simulink model "AOCS system"  (R2023b)
settings: Solver=ode4  StartTime=0.0  StopTime=1000  FixedStep=0.01  RelTol=1e-3
undefined symbols (not defined in the file): A_e, ARW, e_sc, epsilon, H0, J, j_b, k1_slewmanoeuvre, k2_slewmanoeuvre, K_detumbling, Kd, Kp, mu_e, n_sc, n_sun, r_0, R_S2E, Radius_E, RRW, theta0, v_0, w0, w_earth, wnull
libraries: matrix_library x12, vrlib x6, simulink x3, provalibrary x2
settings Model: Creator=alexb  LastModifiedBy=asufx753vdgc013t
settings OptimizationCC: ReuseModelBlockBuffer=off

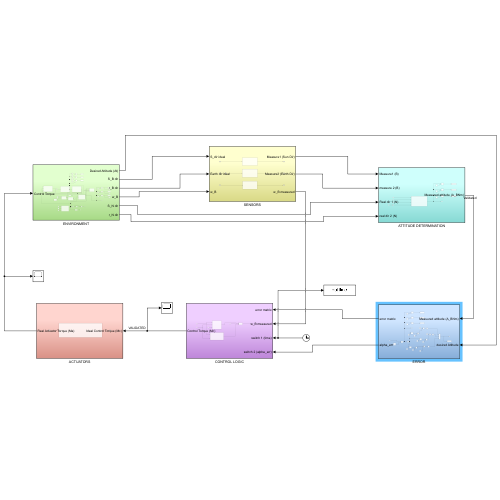
[thumbnail: Simulink's stored preview of the top-level diagram]
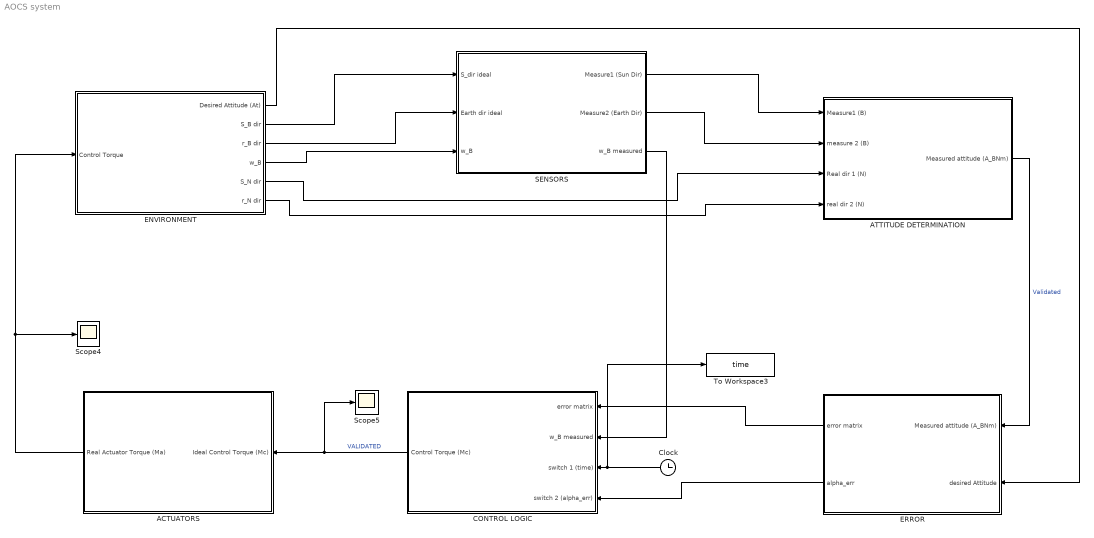
== system AOCS system ==
  ACTUATORS : Subsystem
  ATTITUDE DETERMINATION : Subsystem
  CONTROL LOGIC : Subsystem
  Clock : Clock
  ENVIRONMENT : Subsystem
  ERROR : Subsystem
  SENSORS : Subsystem
  Scope4 : Scope
  Scope5 : Scope
  To Workspace3 : ToWorkspace  VariableName=time  SampleTime=-1
  wires:
  ENVIRONMENT/6(r_N dir) -> ATTITUDE DETERMINATION/4(real dir 2 (N))
  ACTUATORS/1(Real Actuator Torque (Ma)) -> Scope4/1, ENVIRONMENT/1(Control Torque)
  ATTITUDE DETERMINATION/1(Measured attitude (A_BNm)) -> ERROR/1(Measured attitude (A_BNm))  "Validated"
  ENVIRONMENT/3(r_B dir) -> SENSORS/2(Earth dir ideal)
  SENSORS/2(Measure2 (Earth Dir)) -> ATTITUDE DETERMINATION/2(measure 2 (B))
  ENVIRONMENT/1(Desired Attitude (At)) -> ERROR/2(desired Attitude)
  ENVIRONMENT/5(S_N dir) -> ATTITUDE DETERMINATION/3(Real dir 1 (N))
  SENSORS/1(Measure1 (Sun Dir)) -> ATTITUDE DETERMINATION/1(Measure1 (B))
  ENVIRONMENT/2(S_B dir) -> SENSORS/1(S_dir ideal)
  CONTROL LOGIC/1(Control Torque (Mc)) -> Scope5/1, ACTUATORS/1(Ideal Control Torque (Mc))  "VALIDATED"
  ERROR/2(alpha_err) -> CONTROL LOGIC/4(switch 2 (alpha_err))
  ERROR/1(error matrix) -> CONTROL LOGIC/1(error matrix)
  Clock/1 -> To Workspace3/1, CONTROL LOGIC/3(switch 1 (time))
  SENSORS/3(w_B measured) -> CONTROL LOGIC/2(w_B measured)
  ENVIRONMENT/4(w_B) -> SENSORS/3(w_B)

== system AOCS system/ACTUATORS ==
  Ideal Control Torque (Mc) : Inport
  Variable Thrust jets : Subsystem
  Real Actuator Torque (Ma) : Outport
  wires:
  Variable Thrust jets/1(Real Actuator Torque (Ma)) -> Real Actuator Torque (Ma)/1
  Ideal Control Torque (Mc)/1 -> Variable Thrust jets/1(M c)

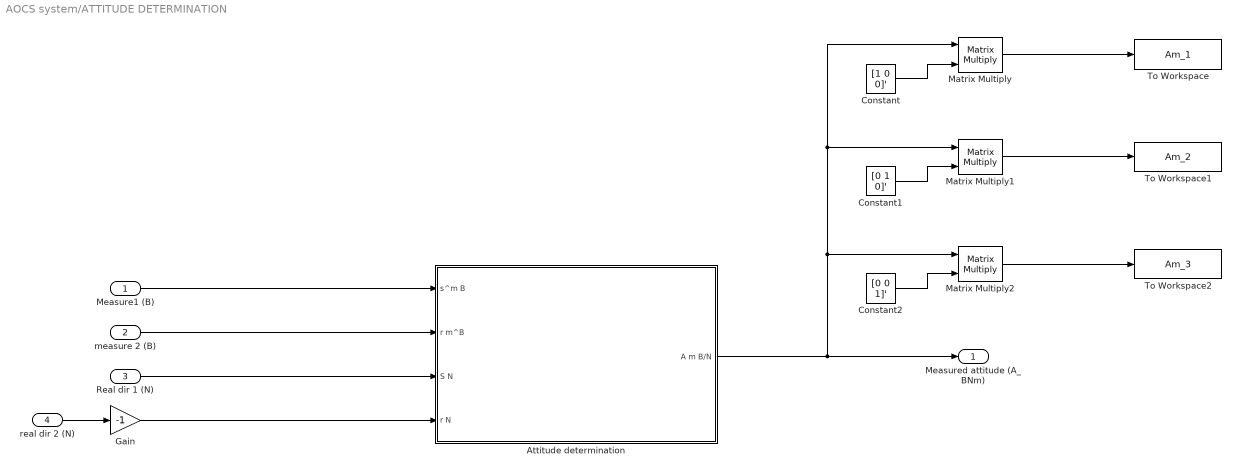
== system AOCS system/ATTITUDE DETERMINATION ==
  Measure1 (B) : Inport
  measure 2 (B) : Inport  Port=2
  Real dir 1 (N) : Inport  Port=3
  real dir 2 (N) : Inport  Port=4
  Attitude determination : Subsystem
  Constant : Constant  Value=[1 0 0]'
  Constant1 : Constant  Value=[0 1 0]'
  Constant2 : Constant  Value=[0 0 1]'
  Gain : Gain  Gain=-1
  Matrix Multiply : Product  Multiplication=Matrix(*)
  Matrix Multiply1 : Product  Multiplication=Matrix(*)
  Matrix Multiply2 : Product  Multiplication=Matrix(*)
  To Workspace : ToWorkspace  VariableName=Am_1  SampleTime=-1
  To Workspace1 : ToWorkspace  VariableName=Am_2  SampleTime=-1
  To Workspace2 : ToWorkspace  VariableName=Am_3  SampleTime=-1
  Measured attitude (A_BNm) : Outport
  wires:
  Measure1 (B)/1 -> Attitude determination/1(s^m B)
  Real dir 1 (N)/1 -> Attitude determination/3(S N)
  real dir 2 (N)/1 -> Gain/1
  measure 2 (B)/1 -> Attitude determination/2(r m^B)
  Gain/1 -> Attitude determination/4(r N)
  Constant/1 -> Matrix Multiply/2
  Matrix Multiply/1 -> To Workspace/1
  Constant1/1 -> Matrix Multiply1/2
  Matrix Multiply1/1 -> To Workspace1/1
  Matrix Multiply2/1 -> To Workspace2/1
  Constant2/1 -> Matrix Multiply2/2
  Attitude determination/1(A m B/N) -> Measured attitude (A_BNm)/1, Matrix Multiply2/1, Matrix Multiply1/1, Matrix Multiply/1

== system AOCS system/CONTROL LOGIC ==
  error matrix : Inport
  w_B measured : Inport  Port=2
  switch 1 (time) : Inport  Port=3
  switch 2 (alpha_err) : Inport  Port=4
  Detumbling and First Slew maneuver : Subsystem
  Nominal Phase Control : Subsystem
  Switch : Switch  Criteria=u2 > Threshold  Threshold=0.3  SaturateOnIntegerOverflow=off  InputSameDT=off
  Control Torque (Mc) : Outport
  wires:
  error matrix/1 -> Detumbling and First Slew maneuver/1(error matrix), Nominal Phase Control/1(error matrix)
  w_B measured/1 -> Detumbling and First Slew maneuver/2(w_B measured), Nominal Phase Control/2(w_B measured)
  switch 1 (time)/1 -> Detumbling and First Slew maneuver/3(switch fucntion 1 (time))
  Nominal Phase Control/1(Control Torque (Mc)) -> Switch/3
  switch 2 (alpha_err)/1 -> Switch/2
  Detumbling and First Slew maneuver/1(Mc) -> Switch/1
  Switch/1 -> Control Torque (Mc)/1

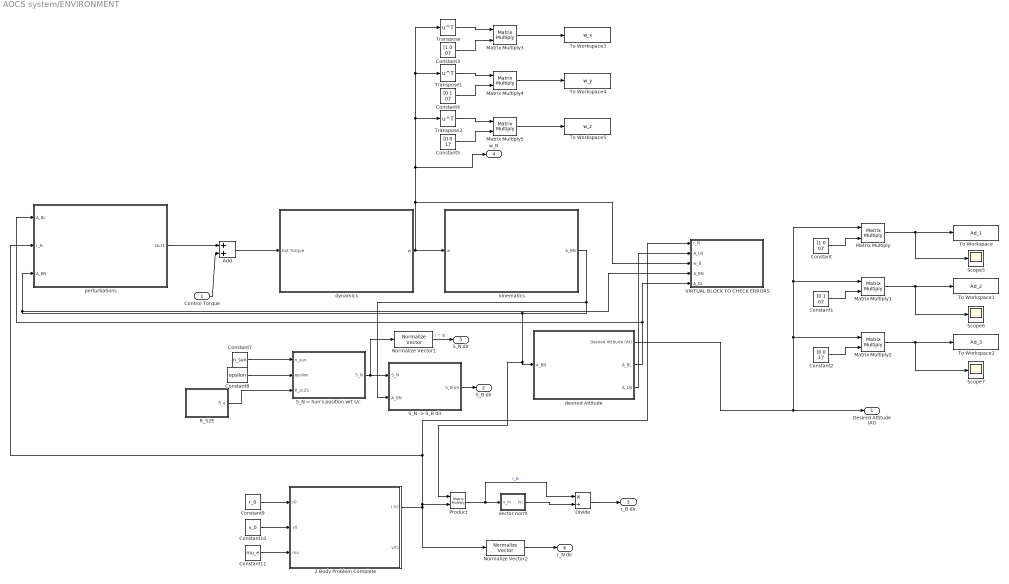
== system AOCS system/ENVIRONMENT ==
  Control Torque : Inport
  2 Body Problem Complete : Subsystem
  Add : Sum
  Constant : Constant  Value=[1 0 0]'
  Constant1 : Constant  Value=[0 1 0]'
  Constant10 : Constant  Value=v_0
  Constant11 : Constant  Value=mu_e
  Constant2 : Constant  Value=[0 0 1]'
  Constant3 : Constant  Value=[1 0 0]'
  Constant4 : Constant  Value=[0 1 0]'
  Constant5 : Constant  Value=[0 0 1]'
  Constant7 : Constant  Value=n_sun
  Constant8 : Constant  Value=epsilon
  Constant9 : Constant  Value=r_0
  Divide : Product  Inputs=*/
  Matrix Multiply{,1..5} (6 alike) : Product  Multiplication=Matrix(*)
  Normalize Vector1 : vrlib/Utilities/Normalize Vector  maxzero=0
  Normalize Vector2 : vrlib/Utilities/Normalize Vector  maxzero=0
  Product : Product  Multiplication=Matrix(*)
  R_S2E : Subsystem
  "S_N -> S_B dir" : Subsystem
  S_N = Sun's position wrt s/c : Subsystem
  Scope5 : Scope
  Scope6 : Scope
  Scope7 : Scope
  To Workspace : ToWorkspace  VariableName=Ad_1  SampleTime=-1
  To Workspace1 : ToWorkspace  VariableName=Ad_2  SampleTime=-1
  To Workspace2 : ToWorkspace  VariableName=Ad_3  SampleTime=-1
  To Workspace3 : ToWorkspace  VariableName=w_x  SampleTime=-1
  To Workspace4 : ToWorkspace  VariableName=w_y  SampleTime=-1
  To Workspace5 : ToWorkspace  VariableName=w_z  SampleTime=-1
  Transpose : Math  Operator=transpose
  Transpose1 : Math  Operator=transpose
  Transpose2 : Math  Operator=transpose
  VIRTUAL BLOCK TO CHECK ERRORS : Subsystem
  "desired Attitude " : Subsystem
  dynamics : Subsystem
  kinematics : Subsystem
  perturbations : Subsystem
  vector norm : Subsystem
  Desired Attitude (At) : Outport
  S_B dir : Outport  Port=2
  r_B dir : Outport  Port=3
  w_B : Outport  Port=4
  S_N dir : Outport  Port=5
  r_N dir : Outport  Port=6
  wires:
  Constant11/1 -> 2 Body Problem Complete/3(mu)
  Constant10/1 -> 2 Body Problem Complete/2(v0)
  Constant9/1 -> 2 Body Problem Complete/1(r0)
  kinematics/1(A_BN) -> "S_N -> S_B dir"/2(A_BN), VIRTUAL BLOCK TO CHECK ERRORS/4(A_BN), perturbations/3(A_BN), Product/1, "desired Attitude "/1(A_BN)
  Control Torque/1 -> Add/2
  Add/1 -> dynamics/1(Ext Torque)
  Constant8/1 -> S_N = Sun's position wrt s/c/2(epsilon)
  R_S2E/1(R_e) -> S_N = Sun's position wrt s/c/3(R_sc2S)
  Constant7/1 -> S_N = Sun's position wrt s/c/1(n_sun)
  S_N = Sun's position wrt s/c/1(S_N) -> Normalize Vector1/1, "S_N -> S_B dir"/1(S_N)
  "S_N -> S_B dir"/1(S_B dir) -> S_B dir/1
  2 Body Problem Complete/1("r (t) ") -> VIRTUAL BLOCK TO CHECK ERRORS/1(r_N), perturbations/2(r_N), Product/2, Normalize Vector2/1
  "desired Attitude "/2(A_BL) -> VIRTUAL BLOCK TO CHECK ERRORS/5(A_BL), perturbations/1(A_BL)
  "desired Attitude "/3(A_LN) -> VIRTUAL BLOCK TO CHECK ERRORS/2(A_LN)
  Product/1 -> Divide/1, vector norm/1(v_in)  "r_B"
  vector norm/1(|v|) -> Divide/2
  Divide/1 -> r_B dir/1
  Normalize Vector1/1 -> S_N dir/1  "r ^ B"
  Normalize Vector2/1 -> r_N dir/1
  perturbations/1(Out1) -> Add/1
  Matrix Multiply/1 -> Scope5/1, To Workspace/1
  Matrix Multiply1/1 -> Scope6/1, To Workspace1/1
  Constant1/1 -> Matrix Multiply1/2
  Constant/1 -> Matrix Multiply/2
  "desired Attitude "/1(Desired Attitude (At)) -> Matrix Multiply2/1, Matrix Multiply1/1, Matrix Multiply/1, Desired Attitude (At)/1
  Constant2/1 -> Matrix Multiply2/2
  Matrix Multiply2/1 -> Scope7/1, To Workspace2/1
  Matrix Multiply3/1 -> To Workspace3/1
  Constant3/1 -> Matrix Multiply3/2
  Transpose/1 -> Matrix Multiply3/1
  Constant4/1 -> Matrix Multiply4/2
  Matrix Multiply4/1 -> To Workspace4/1
  Transpose1/1 -> Matrix Multiply4/1
  dynamics/1(w) -> kinematics/1(w), VIRTUAL BLOCK TO CHECK ERRORS/3(w_B), Transpose2/1, Transpose1/1, Transpose/1, w_B/1
  Matrix Multiply5/1 -> To Workspace5/1
  Constant5/1 -> Matrix Multiply5/2
  Transpose2/1 -> Matrix Multiply5/1

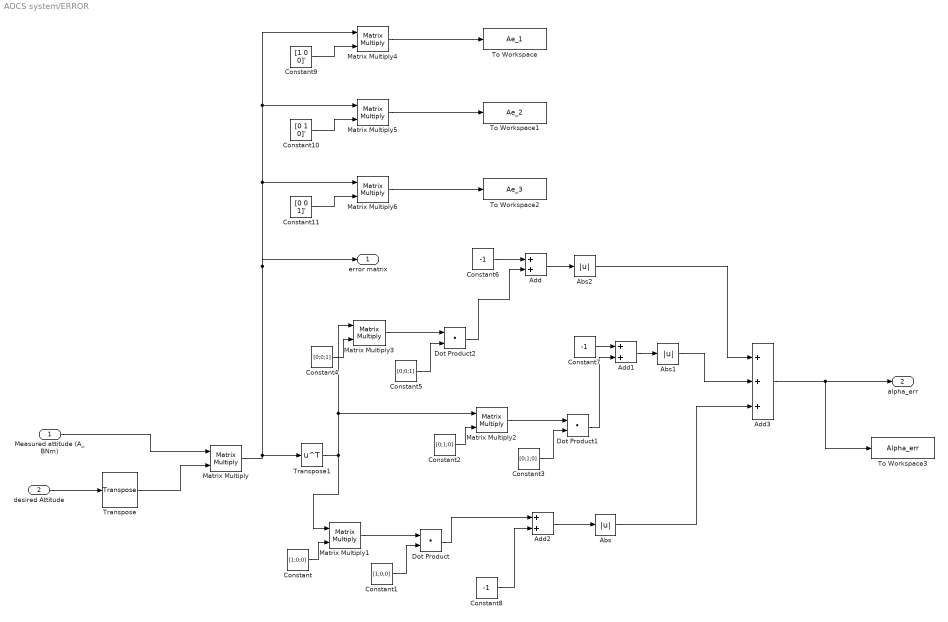
== system AOCS system/ERROR ==
  Measured attitude (A_BNm) : Inport
  desired Attitude : Inport  Port=2
  Abs : Abs  SaturateOnIntegerOverflow=off
  Abs1 : Abs  SaturateOnIntegerOverflow=off
  Abs2 : Abs  SaturateOnIntegerOverflow=off
  Add : Sum
  Add1 : Sum
  Add2 : Sum
  Add3 : Sum  Inputs=+++
  Constant : Constant  Value=[1;0;0]
  Constant1 : Constant  Value=[1;0;0]
  Constant10 : Constant  Value=[0 1 0]'
  Constant11 : Constant  Value=[0 0 1]'
  Constant2 : Constant  Value=[0;1;0]
  Constant3 : Constant  Value=[0;1;0]
  Constant4 : Constant  Value=[0;0;1]
  Constant5 : Constant  Value=[0;0;1]
  Constant6 : Constant  Value=-1
  Constant7 : Constant  Value=-1
  Constant8 : Constant  Value=-1
  Constant9 : Constant  Value=[1 0 0]'
  Dot Product : DotProduct  OutDataTypeStr=Inherit: Inherit via internal rule
  Dot Product1 : DotProduct  OutDataTypeStr=Inherit: Inherit via internal rule
  Dot Product2 : DotProduct  OutDataTypeStr=Inherit: Inherit via internal rule
  Matrix Multiply{,1..6} (7 alike) : Product  Multiplication=Matrix(*)
  To Workspace : ToWorkspace  VariableName=Ae_1  SampleTime=-1
  To Workspace1 : ToWorkspace  VariableName=Ae_2  SampleTime=-1
  To Workspace2 : ToWorkspace  VariableName=Ae_3  SampleTime=-1
  To Workspace3 : ToWorkspace  VariableName=Alpha_err  SampleTime=-1
  Transpose : matrix_library/Transpose
  Transpose1 : Math  Operator=transpose
  error matrix : Outport
  alpha_err : Outport  Port=2
  wires:
  desired Attitude/1 -> Transpose/1
  Measured attitude (A_BNm)/1 -> Matrix Multiply/1
  Transpose/1 -> Matrix Multiply/2
  Matrix Multiply1/1 -> Dot Product/1
  Constant/1 -> Matrix Multiply1/2
  Constant1/1 -> Dot Product/2
  Dot Product/1 -> Add2/1
  Dot Product1/1 -> Add1/2
  Constant2/1 -> Matrix Multiply2/2
  Matrix Multiply2/1 -> Dot Product1/1
  Constant3/1 -> Dot Product1/2
  Dot Product2/1 -> Add/2
  Constant4/1 -> Matrix Multiply3/2
  Matrix Multiply3/1 -> Dot Product2/1
  Constant5/1 -> Dot Product2/2
  Transpose1/1 -> Matrix Multiply1/1, Matrix Multiply2/1, Matrix Multiply3/1
  Constant6/1 -> Add/1
  Constant7/1 -> Add1/1
  Constant8/1 -> Add2/2
  Add2/1 -> Abs/1
  Add1/1 -> Abs1/1
  Add/1 -> Abs2/1
  Abs2/1 -> Add3/1
  Abs1/1 -> Add3/2
  Abs/1 -> Add3/3
  Add3/1 -> To Workspace3/1, alpha_err/1
  Matrix Multiply4/1 -> To Workspace/1
  Matrix Multiply5/1 -> To Workspace1/1
  Constant10/1 -> Matrix Multiply5/2
  Constant9/1 -> Matrix Multiply4/2
  Matrix Multiply/1 -> Transpose1/1, Matrix Multiply6/1, Matrix Multiply5/1, Matrix Multiply4/1, error matrix/1
  Constant11/1 -> Matrix Multiply6/2
  Matrix Multiply6/1 -> To Workspace2/1

== system AOCS system/SENSORS ==
  S_dir ideal : Inport
  Earth dir ideal : Inport  Port=2
  w_B : Inport  Port=3
  Gain : Gain  Gain=-1
  HORIZON SENSOR : Subsystem
  SUN SENSOR : Subsystem
  W sensor (GYRO) : Subsystem
  Measure1 (Sun Dir) : Outport
  Measure2 (Earth Dir) : Outport  Port=2
  w_B measured : Outport  Port=3
  wires:
  SUN SENSOR/1(Sensed S^B) -> Measure1 (Sun Dir)/1  "s^m B"
  S_dir ideal/1 -> SUN SENSOR/1(Real S B)
  Earth dir ideal/1 -> Gain/1
  HORIZON SENSOR/1(Sensed r ^ B1) -> Measure2 (Earth Dir)/1  "r m ^ B"
  Gain/1 -> HORIZON SENSOR/1(Earth dir ideal)
  W sensor (GYRO)/1(w_B measured) -> w_B measured/1
  w_B/1 -> W sensor (GYRO)/1(w_B)

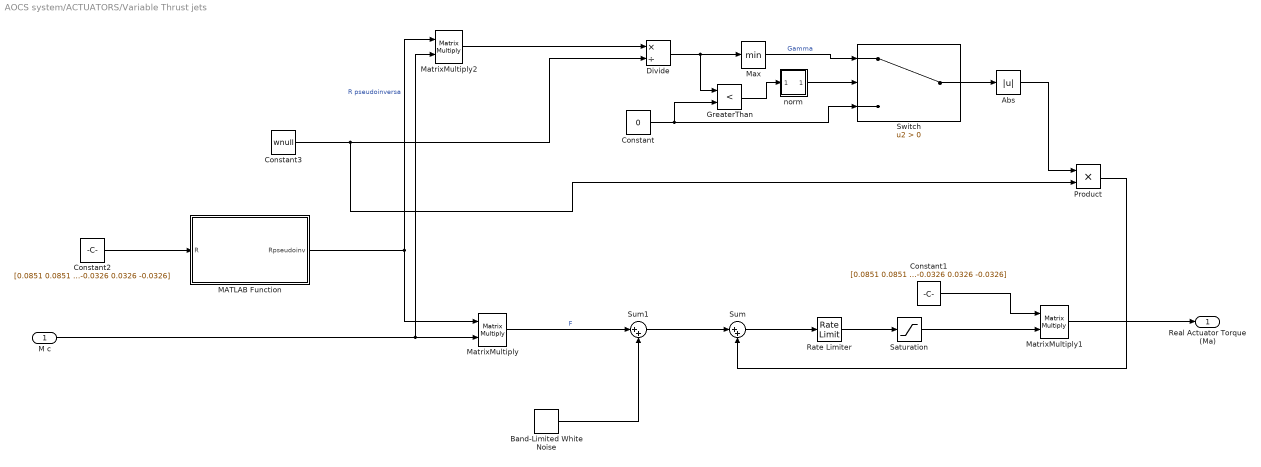
== system AOCS system/ACTUATORS/Variable Thrust jets ==
  M c : Inport
  Abs : Abs  SaturateOnIntegerOverflow=off
  Band-Limited White Noise : simulink/Sources/Band-Limited White Noise  Cov=[0.00001]  Ts=10  seed=[23341]
  Constant : Constant  Value=0
  Constant1 : Constant  Value=[0.0851 0.0851 -0.0851 -0.0851; -0.0525 0.0525 0.0525 -0.0525; 0.0326 -0.0326 0.0326 -0.0326]
  Constant2 : Constant  Value=[0.0851 0.0851 -0.0851 -0.0851; -0.0525 0.0525 0.0525 -0.0525; 0.0326 -0.0326 0.0326 -0.0326]
  Constant3 : Constant  Value=wnull
  Divide : Product  Inputs=*/
  GreaterThan : RelationalOperator  Operator=<  OutDataTypeStr=boolean  RndMeth=Simplest  InputSameDT=off
  MATLAB Function : MATLAB Function  TreatAsAtomicUnit=on
  MatrixMultiply : Product  Multiplication=Matrix(*)
  MatrixMultiply1 : Product  Multiplication=Matrix(*)
  MatrixMultiply2 : Product  Multiplication=Matrix(*)
  Max : MinMax
  Product : Product
  Rate Limiter : RateLimiter  RisingSlewLimit=500  FallingSlewLimit=-500
  Saturation : Saturate  UpperLimit=0.15  LowerLimit=0
  Sum : Sum  Inputs=|++
  Sum1 : Sum  Inputs=|++
  Switch : Switch  Criteria=u2 > Threshold  SaturateOnIntegerOverflow=off  InputSameDT=off
  norm : Subsystem
  Real Actuator Torque (Ma) : Outport
  wires:
  Sum/1 -> Rate Limiter/1
  Rate Limiter/1 -> Saturation/1
  MatrixMultiply1/1 -> Real Actuator Torque (Ma)/1
  Constant2/1 -> MATLAB Function/1(R)
  MatrixMultiply2/1 -> Divide/1
  Divide/1 -> GreaterThan/1, Max/1
  Constant3/1 -> Divide/2, Product/2
  MatrixMultiply/1 -> Sum1/1  "F"
  Sum1/1 -> Sum/1
  Switch/1 -> Abs/1
  Constant/1 -> Switch/3, GreaterThan/2
  Max/1 -> Switch/1  "Gamma"
  GreaterThan/1 -> norm/1(In1)
  norm/1(Out1) -> Switch/2
  M c/1 -> MatrixMultiply2/2, MatrixMultiply/2
  MATLAB Function/1(Rpseudoinv) -> MatrixMultiply2/1, MatrixMultiply/1  "R pseudoinversa"
  Constant1/1 -> MatrixMultiply1/1
  Saturation/1 -> MatrixMultiply1/2
  Abs/1 -> Product/1
  Product/1 -> Sum/2
  Band-Limited White Noise/1 -> Sum1/2

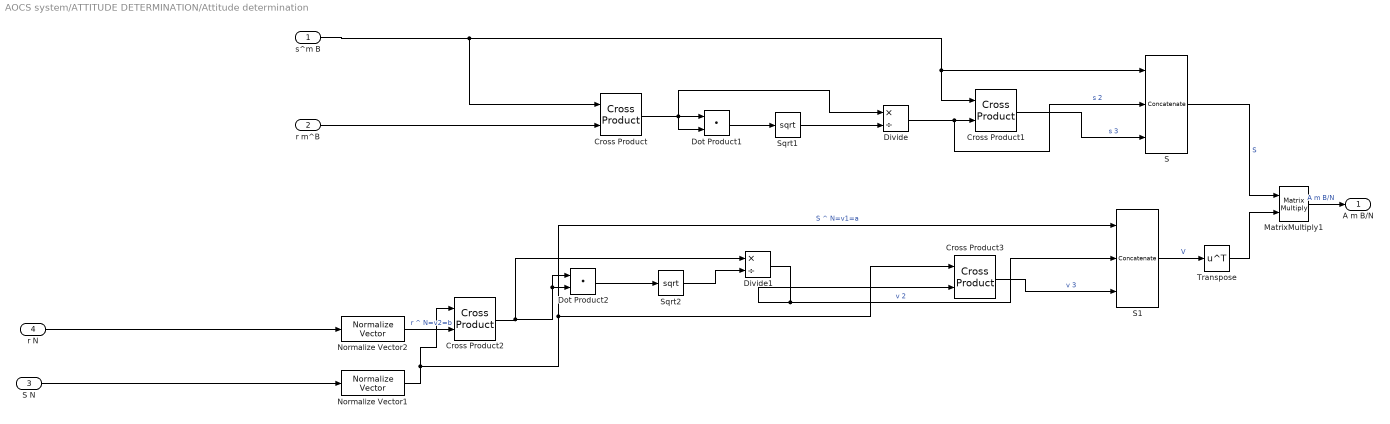
== system AOCS system/ATTITUDE DETERMINATION/Attitude determination ==
  s^m B : Inport
  r m^B : Inport  Port=2
  S N : Inport  Port=3
  r N : Inport  Port=4
  Cross Product{,1..3} (4 alike) : matrix_library/Cross Product
  Divide : Product  Inputs=*/
  Divide1 : Product  Inputs=*/
  Dot Product1 : DotProduct  OutDataTypeStr=Inherit: Inherit via internal rule
  Dot Product2 : DotProduct  OutDataTypeStr=Inherit: Inherit via internal rule
  MatrixMultiply1 : Product  Multiplication=Matrix(*)
  Normalize Vector1 : vrlib/Utilities/Normalize Vector  maxzero=0
  Normalize Vector2 : vrlib/Utilities/Normalize Vector  maxzero=0
  S : Concatenate  NumInputs=3  Mode=Multidimensional array  ConcatenateDimension=2
  S1 : Concatenate  NumInputs=3  Mode=Multidimensional array  ConcatenateDimension=2
  Sqrt1 : Sqrt
  Sqrt2 : Sqrt
  Transpose : Math  Operator=transpose
  A m B/N : Outport
  wires:
  Dot Product1/1 -> Sqrt1/1
  Sqrt2/1 -> Divide1/2
  Cross Product3/1 -> S1/3  "v 3"
  S1/1 -> Transpose/1  "V"
  Divide1/1 -> Cross Product3/2, S1/2  "v 2"
  Cross Product/1 -> Divide/1, Dot Product1/2, Dot Product1/1
  s^m B/1 -> S/1, Cross Product1/1, Cross Product/1
  MatrixMultiply1/1 -> A m B/N/1  "A m B/N"
  Dot Product2/1 -> Sqrt2/1
  Divide/1 -> S/2, Cross Product1/2  "s 2"
  Transpose/1 -> MatrixMultiply1/2
  Normalize Vector1/1 -> Cross Product2/1, S1/1, Cross Product3/1  "S ^ N=v1=a"
  Sqrt1/1 -> Divide/2
  Cross Product1/1 -> S/3  "s 3"
  Normalize Vector2/1 -> Cross Product2/2  "r ^ N=v2=b"
  S/1 -> MatrixMultiply1/1  "S"
  Cross Product2/1 -> Divide1/1, Dot Product2/1, Dot Product2/2
  S N/1 -> Normalize Vector1/1
  r m^B/1 -> Cross Product/2
  r N/1 -> Normalize Vector2/1

== system AOCS system/CONTROL LOGIC/Detumbling and First Slew maneuver ==
  error matrix : Inport
  w_B measured : Inport  Port=2
  switch fucntion 1 (time) : Inport  Port=3
  Detumbling Phase Control : Subsystem
  Slew Maneuver Phase Control : Subsystem
  Switch1 : Switch  Threshold=40  SaturateOnIntegerOverflow=off  InputSameDT=off
  Mc : Outport
  wires:
  w_B measured/1 -> Slew Maneuver Phase Control/2(w_m), Detumbling Phase Control/1(w_measured)
  switch fucntion 1 (time)/1 -> Switch1/2
  Slew Maneuver Phase Control/1(Out1) -> Switch1/1
  Detumbling Phase Control/1(Mc) -> Switch1/3
  Switch1/1 -> Mc/1
  error matrix/1 -> Slew Maneuver Phase Control/1(error matrix)

== system AOCS system/CONTROL LOGIC/Nominal Phase Control ==
  error matrix : Inport
  w_B measured : Inport  Port=2
  Constant : Constant  Value=[0 -1 0; 1 0 0; 0 0 1]
  Control Logic : Subsystem
  Control Torque (Mc) : Outport
  wires:
  w_B measured/1 -> Control Logic/2(w_B measured)
  Constant/1 -> Control Logic/1(A_BL target)
  error matrix/1 -> Control Logic/3(A error)
  Control Logic/1(M c ideal) -> Control Torque (Mc)/1  "M c"

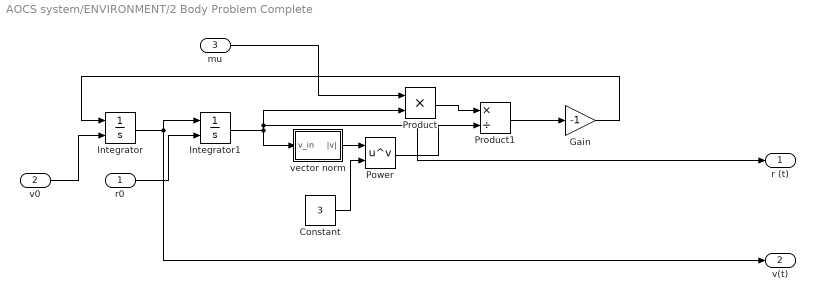
== system AOCS system/ENVIRONMENT/2 Body Problem Complete ==
  r0 : Inport
  v0 : Inport  Port=2
  mu : Inport  Port=3
  Constant : Constant  Value=3
  Gain : Gain  Gain=-1
  Integrator : Integrator  InitialConditionSource=external
  Integrator1 : Integrator  InitialConditionSource=external
  Power : Math  Operator=pow
  Product : Product
  Product1 : Product  Inputs=*/
  vector norm : Subsystem
  "r (t) " : Outport
  v(t) : Outport  Port=2
  wires:
  Integrator/1 -> v(t)/1, Integrator1/1
  v0/1 -> Integrator/2
  r0/1 -> Integrator1/2
  Integrator1/1 -> "r (t) "/1, Product/2, vector norm/1(v_in)
  mu/1 -> Product/1
  Product/1 -> Product1/1
  vector norm/1(|v|) -> Power/1
  Constant/1 -> Power/2
  Power/1 -> Product1/2
  Product1/1 -> Gain/1
  Gain/1 -> Integrator/1

== system AOCS system/ENVIRONMENT/R_S2E ==
  Constant : Constant  Value=R_S2E
  R_e : Outport
  wires:
  Constant/1 -> R_e/1

== system AOCS system/ENVIRONMENT/S_N -> S_B dir ==
  S_N : Inport
  A_BN : Inport  Port=2
  Dot Product : DotProduct  OutDataTypeStr=Inherit: Inherit via internal rule
  Product1 : Product  Multiplication=Matrix(*)
  Product2 : Product  Inputs=*/
  Square Root : Sqrt
  S_B dir : Outport
  wires:
  Product1/1 -> Product2/1, Dot Product/1, Dot Product/2  "S_B"
  Square Root/1 -> Product2/2
  Dot Product/1 -> Square Root/1
  Product2/1 -> S_B dir/1  "Sdir_B"
  S_N/1 -> Product1/2
  A_BN/1 -> Product1/1

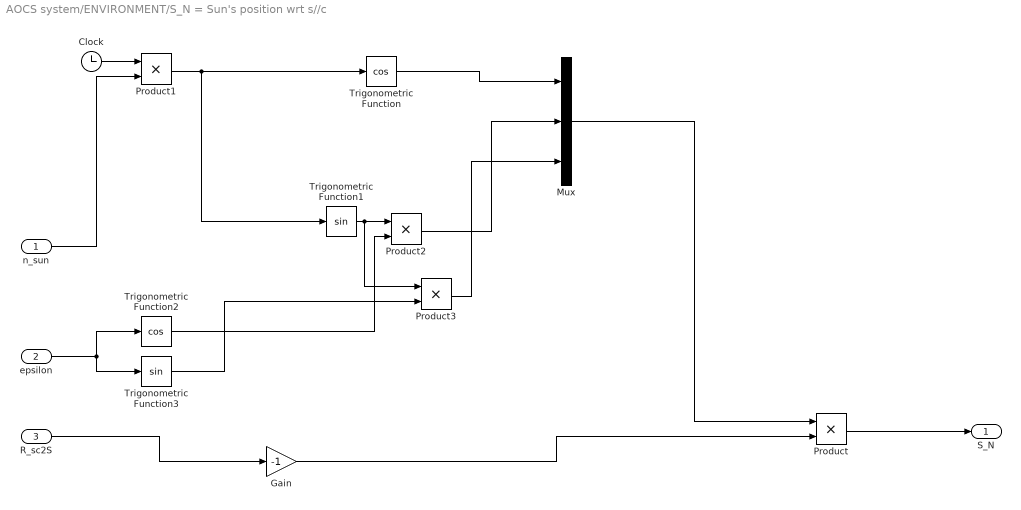
== system AOCS system/ENVIRONMENT/S_N = Sun's position wrt s//c ==
  n_sun : Inport
  epsilon : Inport  Port=2
  R_sc2S : Inport  Port=3
  Clock : Clock
  Gain : Gain  Gain=-1
  Mux : Mux  Inputs=3
  Product{,1..3} (4 alike) : Product
  Trigonometric Function : Trigonometry  Operator=cos
  Trigonometric Function1 : Trigonometry
  Trigonometric Function2 : Trigonometry  Operator=cos
  Trigonometric Function3 : Trigonometry
  S_N : Outport
  wires:
  Clock/1 -> Product1/1
  n_sun/1 -> Product1/2
  Product1/1 -> Trigonometric Function1/1, Trigonometric Function/1
  Trigonometric Function1/1 -> Product3/1, Product2/1
  epsilon/1 -> Trigonometric Function3/1, Trigonometric Function2/1
  Trigonometric Function2/1 -> Product2/2
  Trigonometric Function3/1 -> Product3/2
  Trigonometric Function/1 -> Mux/1
  Product2/1 -> Mux/2
  Product3/1 -> Mux/3
  Mux/1 -> Product/1
  Product/1 -> S_N/1
  R_sc2S/1 -> Gain/1
  Gain/1 -> Product/2

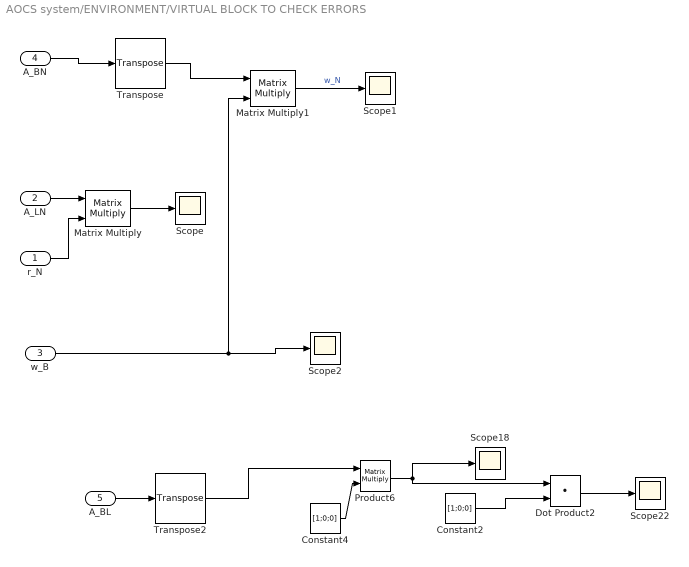
== system AOCS system/ENVIRONMENT/VIRTUAL BLOCK TO CHECK ERRORS ==
  r_N : Inport
  A_LN : Inport  Port=2
  w_B : Inport  Port=3
  A_BN : Inport  Port=4
  A_BL : Inport  Port=5
  Constant2 : Constant  Value=[1;0;0]
  Constant4 : Constant  Value=[1;0;0]
  Dot Product2 : DotProduct  OutDataTypeStr=Inherit: Inherit via internal rule
  Matrix Multiply : Product  Multiplication=Matrix(*)
  Matrix Multiply1 : Product  Multiplication=Matrix(*)
  Product6 : Product  Multiplication=Matrix(*)
  Scope{,1..2,18,22} (5 alike) : Scope
  Transpose : matrix_library/Transpose
  Transpose2 : matrix_library/Transpose
  wires:
  A_LN/1 -> Matrix Multiply/1
  r_N/1 -> Matrix Multiply/2
  Matrix Multiply/1 -> Scope/1
  A_BN/1 -> Transpose/1
  Transpose/1 -> Matrix Multiply1/1
  w_B/1 -> Scope2/1, Matrix Multiply1/2
  Matrix Multiply1/1 -> Scope1/1  "w_N"
  Constant4/1 -> Product6/2
  Constant2/1 -> Dot Product2/2
  Dot Product2/1 -> Scope22/1
  Transpose2/1 -> Product6/1
  Product6/1 -> Dot Product2/1, Scope18/1
  A_BL/1 -> Transpose2/1

== system AOCS system/ENVIRONMENT/desired Attitude  ==
  A_BN : Inport
  2 Body Probelm : Subsystem
  A_BL determination : Subsystem
  Constant3 : Constant  Value=theta0
  Constant5 : Constant  Value=e_sc
  Constant6 : Constant  Value=n_sc
  Subsystem3 : Subsystem
  Desired Attitude (At) : Outport
  A_BL : Outport  Port=2
  A_LN : Outport  Port=3
  wires:
  Constant6/1 -> 2 Body Probelm/3(n_sc)
  Constant3/1 -> 2 Body Probelm/2(theta0)
  Constant5/1 -> 2 Body Probelm/1(e_sc)
  2 Body Probelm/1(theta_sc) -> A_BL determination/2(theta)
  A_BN/1 -> A_BL determination/1(A_BN)
  A_BL determination/1(A_BL) -> A_BL/1  "A_BL"
  A_BL determination/2(A_LN) -> A_LN/1, Subsystem3/1(A L/N)
  Subsystem3/1(Desired Attitude (At)) -> Desired Attitude (At)/1

== system AOCS system/ENVIRONMENT/dynamics ==
  Ext Torque : Inport
  Constant : Constant  Value=J
  Constant1 : Constant  Value=w0
  "Dynamic solver Perturbed (J, w_0, M_ext)" : Subsystem
  w : Outport
  wires:
  Constant/1 -> "Dynamic solver Perturbed (J, w_0, M_ext)"/1(J)
  Constant1/1 -> "Dynamic solver Perturbed (J, w_0, M_ext)"/2(w0)
  Ext Torque/1 -> "Dynamic solver Perturbed (J, w_0, M_ext)"/3(External Torque)
  "Dynamic solver Perturbed (J, w_0, M_ext)"/1(w) -> w/1

== system AOCS system/ENVIRONMENT/kinematics ==
  w : Inport
  w(t) to DirectorCosines : provalibrary/w(t) to DirectorCosines  SystemSampleTime=-1  VariantActivationTime=update diagram  AllowFlexibleInterface=on  Latency=0  AutoFrameSizeCalculation=off
  A_BN : Outport
  wires:
  w/1 -> w(t) to DirectorCosines/1
  w(t) to DirectorCosines/1 -> A_BN/1

== system AOCS system/ENVIRONMENT/perturbations ==
  A_BL : Inport
  r_N : Inport  Port=2
  A_BN : Inport  Port=3
  Add : Sum
  Constant : Constant  Value=J
  Gravity Gradient Torque (GTT) : Subsystem
  Magnetic Torque (temporary) : Subsystem
  vector norm : Subsystem
  vector norm1 : Subsystem
  Out1 : Outport
  wires:
  Constant/1 -> Gravity Gradient Torque (GTT)/1(J)
  A_BL/1 -> Gravity Gradient Torque (GTT)/2(A_BL)
  r_N/1 -> Magnetic Torque (temporary)/1(r_N)
  A_BN/1 -> Magnetic Torque (temporary)/2(A_BN)
  Gravity Gradient Torque (GTT)/1(v_in) -> vector norm/1(v_in), Add/1
  Magnetic Torque (temporary)/1(Magnetic Torque) -> Add/2, vector norm1/1(v_in)
  Add/1 -> Out1/1

== system AOCS system/ENVIRONMENT/vector norm ==
  v_in : Inport
  Dot Product : DotProduct  OutDataTypeStr=Inherit: Inherit via internal rule
  Square Root : Sqrt
  |v| : Outport
  wires:
  v_in/1 -> Dot Product/2, Dot Product/1
  Dot Product/1 -> Square Root/1
  Square Root/1 -> |v|/1

== system AOCS system/SENSORS/HORIZON SENSOR ==
  Earth dir ideal : Inport
  Constant : Constant  Value=0.166
  MATLAB Function : MATLAB Function  TreatAsAtomicUnit=on
  Matrix Multiply : Product  Multiplication=Matrix(*)
  Normalize Vector1 : vrlib/Utilities/Normalize Vector  maxzero=0
  Sensed r ^ B : Subsystem
  Sensed r ^ B1 : Outport
  wires:
  Sensed r ^ B/1(Sensed r ^ B) -> Sensed r ^ B1/1  "Sensed r ^ B"
  Normalize Vector1/1 -> Sensed r ^ B/1(In1)  "r ^ B"
  Earth dir ideal/1 -> Matrix Multiply/2
  MATLAB Function/1(y) -> Matrix Multiply/1
  Constant/1 -> MATLAB Function/1(u)
  Matrix Multiply/1 -> Normalize Vector1/1

== system AOCS system/SENSORS/SUN SENSOR ==
  Real S B : Inport
  Constant : Constant  Value=0.02
  MATLAB Function : MATLAB Function  TreatAsAtomicUnit=on
  Matrix Multiply : Product  Multiplication=Matrix(*)
  Normalize Vector1 : vrlib/Utilities/Normalize Vector  maxzero=0
  Sensed S^ B x : Subsystem
  Sensed S^B : Outport
  wires:
  Real S B/1 -> Matrix Multiply/2  "S B"
  Sensed S^ B x/1(Sensed S B) -> Sensed S^B/1  "Sensed S^ B"
  Normalize Vector1/1 -> Sensed S^ B x/1(In1)
  Matrix Multiply/1 -> Normalize Vector1/1
  MATLAB Function/1(y) -> Matrix Multiply/1
  Constant/1 -> MATLAB Function/1(u)

== system AOCS system/SENSORS/W sensor (GYRO) ==
  w_B : Inport
  Add : Sum  Inputs=+++
  Constant : Constant  Value=RRW
  Constant1 : Constant  Value=ARW
  Constant2 : Constant  Value=A_e  VectorParams1D=off
  Matrix Multiply : Product  Multiplication=Matrix(*)
  w_B measured : Outport
  wires:
  Constant1/1 -> Add/2
  Constant/1 -> Add/3
  Add/1 -> w_B measured/1
  Matrix Multiply/1 -> Add/1
  w_B/1 -> Matrix Multiply/2
  Constant2/1 -> Matrix Multiply/1

== system AOCS system/ACTUATORS/Variable Thrust jets/norm ==
  In1 : Inport
  Dot Product : DotProduct  OutDataTypeStr=Inherit: Inherit via internal rule
  Sqrt : Sqrt
  Out1 : Outport
  wires:
  In1/1 -> Dot Product/2, Dot Product/1
  Dot Product/1 -> Sqrt/1
  Sqrt/1 -> Out1/1

== system AOCS system/CONTROL LOGIC/Detumbling and First Slew maneuver/Detumbling Phase Control ==
  w_measured : Inport
  Gain : Gain  Gain=-K_detumbling
  Mc : Outport
  wires:
  w_measured/1 -> Gain/1
  Gain/1 -> Mc/1

== system AOCS system/CONTROL LOGIC/Detumbling and First Slew maneuver/Slew Maneuver Phase Control ==
  error matrix : Inport
  w_m : Inport  Port=2
  Constant : Constant  Value=J
  Cross Product : matrix_library/Cross Product
  Gain : Gain  Gain=-k2_slewmanoeuvre
  Gain1 : Gain  Gain=-k1_slewmanoeuvre
  MATLAB Function : MATLAB Function  TreatAsAtomicUnit=on
  Matrix Multiply : Product  Multiplication=Matrix(*)
  Sum : Sum  Inputs=|+-
  Sum1 : Sum  Inputs=+++
  Transpose : Math  Operator=transpose
  Out1 : Outport
  wires:
  Sum1/1 -> Out1/1  "M c slew manoeuvre"
  Constant/1 -> Matrix Multiply/1
  w_m/1 -> Matrix Multiply/2, Cross Product/1, Gain1/1
  Gain/1 -> Sum1/1
  Gain1/1 -> Sum1/2
  Cross Product/1 -> Sum1/3
  error matrix/1 -> Sum/2, Transpose/1
  Matrix Multiply/1 -> Cross Product/2
  MATLAB Function/1(vector) -> Gain/1
  Sum/1 -> MATLAB Function/1(u)
  Transpose/1 -> Sum/1

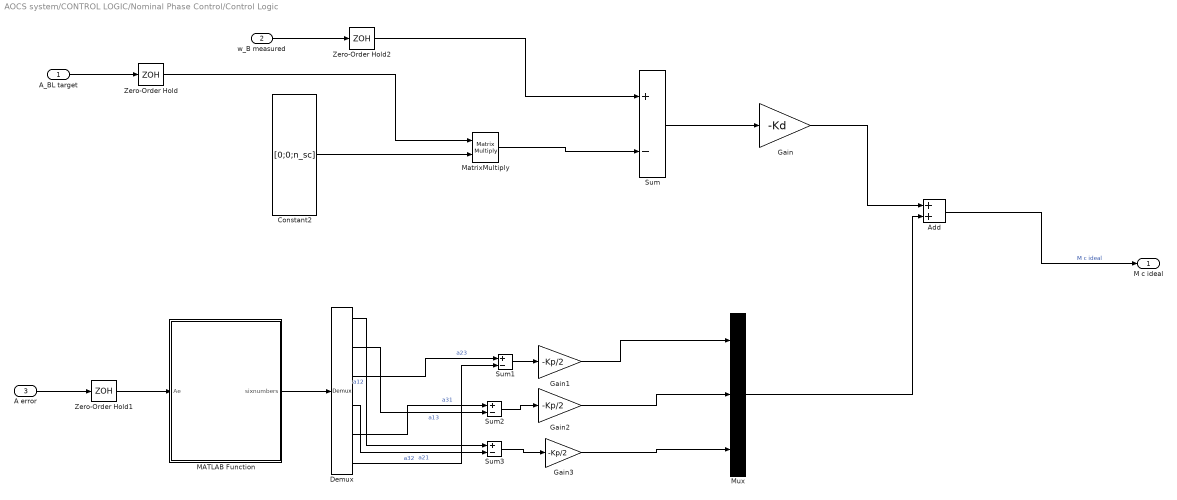
== system AOCS system/CONTROL LOGIC/Nominal Phase Control/Control Logic ==
  A_BL target : Inport
  w_B measured : Inport  Port=2
  A error : Inport  Port=3
  Add : Sum
  Constant2 : Constant  Value=[0;0;n_sc]  VectorParams1D=off
  Demux : Demux  Outputs=6
  Gain : Gain  Gain=-Kd
  Gain1 : Gain  Gain=-Kp/2
  Gain2 : Gain  Gain=-Kp/2
  Gain3 : Gain  Gain=-Kp/2
  MATLAB Function : MATLAB Function  TreatAsAtomicUnit=on
  MatrixMultiply : Product  Multiplication=Matrix(*)
  Mux : Mux  Inputs=3
  Sum{,1..3} (4 alike) : Sum  Inputs=+-
  Zero-Order Hold : ZeroOrderHold  SampleTime=0.02
  Zero-Order Hold1 : ZeroOrderHold  SampleTime=0.02
  Zero-Order Hold2 : ZeroOrderHold  SampleTime=0.02
  M c ideal : Outport
  wires:
  Sum/1 -> Gain/1
  MATLAB Function/1(sixnumbers) -> Demux/1
  Sum2/1 -> Gain2/1
  Demux/5 -> Sum2/1  "a31"
  Sum1/1 -> Gain1/1
  Gain/1 -> Add/1
  Gain2/1 -> Mux/2
  Sum3/1 -> Gain3/1
  Demux/3 -> Sum1/1  "a23"
  Demux/4 -> Sum3/2  "a21"
  Demux/2 -> Sum2/2  "a13"
  Demux/6 -> Sum1/2  "a32"
  Gain1/1 -> Mux/1
  Constant2/1 -> MatrixMultiply/2
  MatrixMultiply/1 -> Sum/2
  Demux/1 -> Sum3/1  "a12"
  Mux/1 -> Add/2
  Add/1 -> M c ideal/1  "M c ideal"
  w_B measured/1 -> Zero-Order Hold2/1
  Gain3/1 -> Mux/3
  A_BL target/1 -> Zero-Order Hold/1
  A error/1 -> Zero-Order Hold1/1
  Zero-Order Hold1/1 -> MATLAB Function/1(Ae)
  Zero-Order Hold/1 -> MatrixMultiply/1
  Zero-Order Hold2/1 -> Sum/1

== system AOCS system/ENVIRONMENT/2 Body Problem Complete/vector norm ==
  v_in : Inport
  Dot Product : DotProduct  OutDataTypeStr=Inherit: Inherit via internal rule
  Square Root : Sqrt
  |v| : Outport
  wires:
  v_in/1 -> Dot Product/2, Dot Product/1
  Dot Product/1 -> Square Root/1
  Square Root/1 -> |v|/1

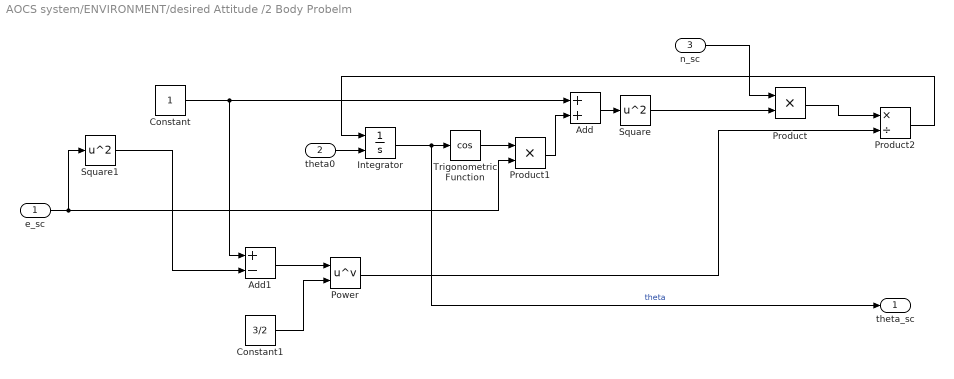
== system AOCS system/ENVIRONMENT/desired Attitude /2 Body Probelm ==
  e_sc : Inport
  theta0 : Inport  Port=2
  n_sc : Inport  Port=3
  Add : Sum
  Add1 : Sum  Inputs=+-
  Constant : Constant
  Constant1 : Constant  Value=3/2
  Integrator : Integrator  InitialConditionSource=external
  Power : Math  Operator=pow
  Product : Product
  Product1 : Product
  Product2 : Product  Inputs=*/
  Square : Math  Operator=square
  Square1 : Math  Operator=square
  Trigonometric Function : Trigonometry  Operator=cos
  theta_sc : Outport
  wires:
  theta0/1 -> Integrator/2
  n_sc/1 -> Product/1
  Constant/1 -> Add1/1, Add/1
  Integrator/1 -> theta_sc/1, Trigonometric Function/1  "theta"
  Trigonometric Function/1 -> Product1/1
  e_sc/1 -> Square1/1, Product1/2
  Product1/1 -> Add/2
  Add/1 -> Square/1
  Square/1 -> Product/2
  Square1/1 -> Add1/2
  Product/1 -> Product2/1
  Add1/1 -> Power/1
  Constant1/1 -> Power/2
  Power/1 -> Product2/2
  Product2/1 -> Integrator/1

== system AOCS system/ENVIRONMENT/desired Attitude /A_BL determination ==
  A_BN : Inport
  theta : Inport  Port=2
  A_LN Definition : Subsystem
  Product1 : Product  Multiplication=Matrix(*)
  Transpose : matrix_library/Transpose
  A_BL : Outport
  A_LN : Outport  Port=2
  wires:
  Product1/1 -> A_BL/1  "A_BL"
  Transpose/1 -> Product1/2
  A_BN/1 -> Product1/1
  theta/1 -> A_LN Definition/1(theta)
  A_LN Definition/1(out) -> A_LN/1, Transpose/1

== system AOCS system/ENVIRONMENT/desired Attitude /Subsystem3 ==
  A L/N : Inport
  A B/L target : Constant  Value=[1 0 0; 0 1 0; 0 0 1]
  MatrixMultiply : Product  Multiplication=Matrix(*)
  Desired Attitude (At) : Outport
  wires:
  MatrixMultiply/1 -> Desired Attitude (At)/1
  A B/L target/1 -> MatrixMultiply/1
  A L/N/1 -> MatrixMultiply/2

== system AOCS system/ENVIRONMENT/dynamics/Dynamic solver Perturbed (J, w_0, M_ext) ==
  J : Inport
  w0 : Inport  Port=2
  External Torque : Inport  Port=3
  Add : Sum
  Cross Product : matrix_library/Cross Product
  Integrator : Integrator  InitialConditionSource=external
  Product : Product  Inputs=/  Multiplication=Matrix(*)
  Product1 : Product  Multiplication=Matrix(*)
  Product2 : Product  Multiplication=Matrix(*)
  vector norm : Subsystem
  w : Outport
  wires:
  Product2/1 -> Integrator/1
  Integrator/1 -> w/1, Cross Product/2, Product1/2  "w"
  J/1 -> Product1/1, Product/1  "J"
  Product1/1 -> vector norm/1(v_in), Cross Product/1  "J * w"
  w0/1 -> Integrator/2
  Product/1 -> Product2/1
  Cross Product/1 -> Add/1
  Add/1 -> Product2/2
  External Torque/1 -> Add/2

== system AOCS system/ENVIRONMENT/perturbations/Gravity Gradient Torque (GTT) ==
  J : Inport
  A_BL : Inport  Port=2
  Constant : Constant  Value=[1;0;0]
  Cross Product1 : matrix_library/Cross Product
  Gain : Gain  Gain=-3 * (n_sc)^2
  Product3 : Product  Multiplication=Matrix(*)
  Product4 : Product  Multiplication=Matrix(*)
  v_in : Outport
  wires:
  J/1 -> Product4/1
  Constant/1 -> Product3/2
  Product3/1 -> Cross Product1/2, Product4/2  "c"
  Product4/1 -> Cross Product1/1  "J * c"
  Cross Product1/1 -> Gain/1
  A_BL/1 -> Product3/1
  Gain/1 -> v_in/1

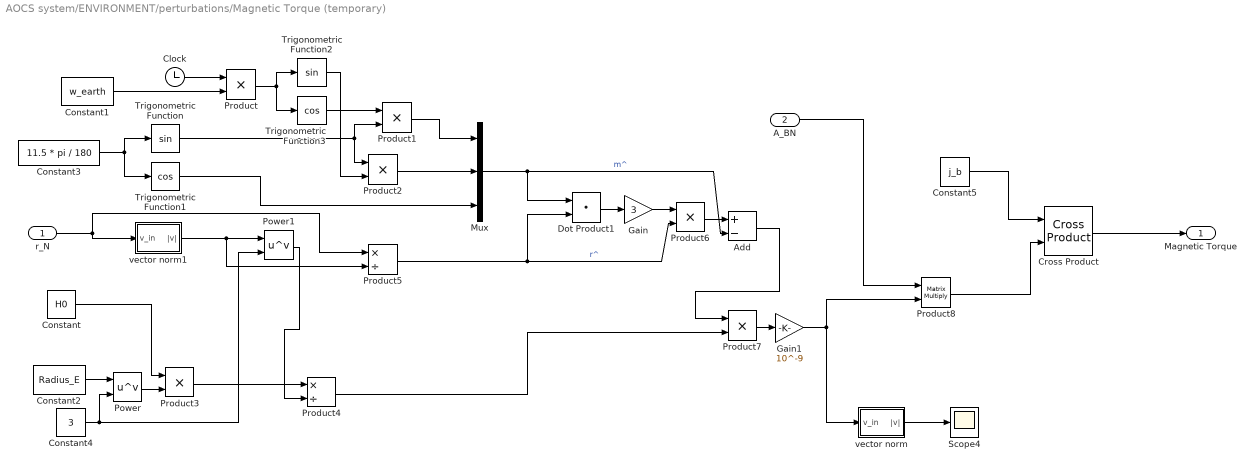
== system AOCS system/ENVIRONMENT/perturbations/Magnetic Torque (temporary) ==
  r_N : Inport
  A_BN : Inport  Port=2
  Add : Sum  Inputs=+-
  Clock : Clock
  Constant : Constant  Value=H0
  Constant1 : Constant  Value=w_earth
  Constant2 : Constant  Value=Radius_E
  Constant3 : Constant  Value=11.5 * pi / 180
  Constant4 : Constant  Value=3
  Constant5 : Constant  Value=j_b
  Cross Product : matrix_library/Cross Product
  Dot Product1 : DotProduct  OutDataTypeStr=Inherit: Inherit via internal rule
  Gain : Gain  Gain=3
  Gain1 : Gain  Gain=10^-9
  Mux : Mux  Inputs=3
  Power : Math  Operator=pow
  Power1 : Math  Operator=pow
  Product{,1..3,6..7} (6 alike) : Product
  Product4 : Product  Inputs=*/
  Product5 : Product  Inputs=*/
  Product8 : Product  Multiplication=Matrix(*)
  Scope4 : Scope
  Trigonometric Function : Trigonometry
  Trigonometric Function1 : Trigonometry  Operator=cos
  Trigonometric Function2 : Trigonometry
  Trigonometric Function3 : Trigonometry  Operator=cos
  vector norm : Subsystem
  vector norm1 : Subsystem
  Magnetic Torque : Outport
  wires:
  r_N/1 -> vector norm1/1(v_in), Product5/1
  Constant3/1 -> Trigonometric Function/1, Trigonometric Function1/1
  Clock/1 -> Product/1
  Constant1/1 -> Product/2
  Product/1 -> Trigonometric Function3/1, Trigonometric Function2/1
  Trigonometric Function3/1 -> Product1/1
  Trigonometric Function/1 -> Product2/1, Product1/2
  Product1/1 -> Mux/1
  Product2/1 -> Mux/2
  Trigonometric Function2/1 -> Product2/2
  Trigonometric Function1/1 -> Mux/3
  Constant2/1 -> Power/1
  Constant4/1 -> Power1/2, Power/2
  Power/1 -> Product3/2
  Constant/1 -> Product3/1
  Product3/1 -> Product4/1
  vector norm1/1(|v|) -> Product5/2, Power1/1
  Power1/1 -> Product4/2
  Mux/1 -> Add/2, Dot Product1/1  "m^"
  Product5/1 -> Product6/2, Dot Product1/2  "r^"
  Dot Product1/1 -> Gain/1
  Gain/1 -> Product6/1
  Product6/1 -> Add/1
  Add/1 -> Product7/1
  Product4/1 -> Product7/2
  Constant5/1 -> Cross Product/1
  Gain1/1 -> vector norm/1(v_in), Product8/2
  vector norm/1(|v|) -> Scope4/1
  Cross Product/1 -> Magnetic Torque/1
  A_BN/1 -> Product8/1
  Product8/1 -> Cross Product/2
  Product7/1 -> Gain1/1

== system AOCS system/ENVIRONMENT/perturbations/vector norm ==
  v_in : Inport
  Dot Product : DotProduct  OutDataTypeStr=Inherit: Inherit via internal rule
  Square Root : Sqrt
  |v| : Outport
  wires:
  v_in/1 -> Dot Product/2, Dot Product/1
  Dot Product/1 -> Square Root/1
  Square Root/1 -> |v|/1

== system AOCS system/ENVIRONMENT/perturbations/vector norm1 ==
  v_in : Inport
  Dot Product : DotProduct  OutDataTypeStr=Inherit: Inherit via internal rule
  Square Root : Sqrt
  |v| : Outport
  wires:
  v_in/1 -> Dot Product/2, Dot Product/1
  Dot Product/1 -> Square Root/1
  Square Root/1 -> |v|/1

== system AOCS system/SENSORS/HORIZON SENSOR/Sensed r ^ B ==
  In1 : Inport
  Band-Limited White Noise : simulink/Sources/Band-Limited White Noise  Cov=[0.00001]  Ts=0.1  seed=[23350]
  Sum : Sum  Inputs=|++
  Zero-Order Hold : ZeroOrderHold  SampleTime=0.1
  Sensed r ^ B : Outport
  wires:
  Sum/1 -> Sensed r ^ B/1  "Sensed r ^ B"
  Zero-Order Hold/1 -> Sum/1
  In1/1 -> Zero-Order Hold/1
  Band-Limited White Noise/1 -> Sum/2

== system AOCS system/SENSORS/SUN SENSOR/Sensed S^ B x ==
  In1 : Inport
  Band-Limited White Noise : simulink/Sources/Band-Limited White Noise  Cov=[0.00001]  Ts=0.1  seed=[23341]
  Sum : Sum  Inputs=|++
  Zero-Order Hold : ZeroOrderHold  SampleTime=0.1
  Sensed S B : Outport
  wires:
  Sum/1 -> Sensed S B/1  "Sensed S B"
  Zero-Order Hold/1 -> Sum/1
  In1/1 -> Zero-Order Hold/1
  Band-Limited White Noise/1 -> Sum/2

== system AOCS system/ENVIRONMENT/desired Attitude /A_BL determination/A_LN Definition ==
  theta : Inport
  Constant : Constant
  Constant1 : Constant  Value=0
  Gain : Gain  Gain=-1
  Trigonometric Function : Trigonometry
  Trigonometric Function1 : Trigonometry  Operator=cos
  comp2matrix3x3 : provalibrary/comp2matrix3x3  SystemSampleTime=-1  VariantActivationTime=update diagram  AllowFlexibleInterface=on  Latency=0  AutoFrameSizeCalculation=off
  out : Outport
  wires:
  theta/1 -> Trigonometric Function/1, Trigonometric Function1/1
  Constant1/1 -> comp2matrix3x3/9, comp2matrix3x3/6, comp2matrix3x3/2, comp2matrix3x3/1
  Constant/1 -> comp2matrix3x3/3
  Trigonometric Function1/1 -> comp2matrix3x3/8, comp2matrix3x3/4
  Trigonometric Function/1 -> comp2matrix3x3/7, Gain/1
  Gain/1 -> comp2matrix3x3/5
  comp2matrix3x3/1 -> out/1

== system AOCS system/ENVIRONMENT/dynamics/Dynamic solver Perturbed (J, w_0, M_ext)/vector norm ==
  v_in : Inport
  Dot Product : DotProduct  OutDataTypeStr=Inherit: Inherit via internal rule
  Square Root : Sqrt
  |v| : Outport
  wires:
  v_in/1 -> Dot Product/2, Dot Product/1
  Dot Product/1 -> Square Root/1
  Square Root/1 -> |v|/1

== system AOCS system/ENVIRONMENT/perturbations/Magnetic Torque (temporary)/vector norm ==
  v_in : Inport
  Dot Product : DotProduct  OutDataTypeStr=Inherit: Inherit via internal rule
  Square Root : Sqrt
  |v| : Outport
  wires:
  v_in/1 -> Dot Product/2, Dot Product/1
  Dot Product/1 -> Square Root/1
  Square Root/1 -> |v|/1

== system AOCS system/ENVIRONMENT/perturbations/Magnetic Torque (temporary)/vector norm1 ==
  v_in : Inport
  Dot Product : DotProduct  OutDataTypeStr=Inherit: Inherit via internal rule
  Square Root : Sqrt
  |v| : Outport
  wires:
  v_in/1 -> Dot Product/2, Dot Product/1
  Dot Product/1 -> Square Root/1
  Square Root/1 -> |v|/1

== matlab function AOCS system/CONTROL LOGIC/Nominal Phase Control/Control Logic/MATLAB Function ==
  data: Ae input; sixnumbers output
function sixnumbers = fcn(Ae)
a12=Ae(1,2);
a13=Ae(1,3);
a21=Ae(2,1);
a31=Ae(3,1);
a32=Ae(3,2);
a23=Ae(2,3);
sixnumbers=[a12;a13;a23;a21;a31;a32];
end

== matlab function AOCS system/CONTROL LOGIC/Detumbling and First Slew maneuver/Slew Maneuver Phase Control/MATLAB Function ==
  data: u input; vector output
function vector = fcn(u)
ax=u(3,2);
ay=u(1,3);
az=u(2,1);
vector=[ax;ay;az];
end

== matlab function AOCS system/SENSORS/SUN SENSOR/MATLAB Function ==
  data: u input; y output
function y = fcn(u)

A_eps = eye(3) - [0, -u * pi / 180, u * pi / 180; u * pi / 180, 0, -u * pi / 180; -u * pi / 180, u * pi / 180, 0];

y = A_eps;


end

== matlab function AOCS system/SENSORS/HORIZON SENSOR/MATLAB Function ==
  data: u input; y output
function y = fcn(u)

A_eps = eye(3) - [0, -u * pi / 180, u * pi / 180; u * pi / 180, 0, -u * pi / 180; -u * pi / 180, u * pi / 180, 0];

y = A_eps;


end

== matlab function AOCS system/ACTUATORS/Variable Thrust jets/MATLAB Function ==
  data: R input; Rpseudoinv output
function Rpseudoinv = fcn(R)
Rpseudoinv=pinv(R);
end
